simulink model "grzej_ret"  (R2019a)
settings: Solver=VariableStepAuto  StartTime=0.0  StopTime=TS  RelTol=1e-3
values from neighbouring files (symbols this model uses):
  cpw = 4175    [LAB1.m]    (also in LAB2.m; LAB3.m)
  Cvg1 = cpw * row * Vg    (= 60120)    [LAB3.m]
  Cvk = Cvg    (= 40080000)    [LAB2.m]    (also in LAB3.m = 4175000; bezp.m = 4163040.816; budynek_z_hydraulika_symulacja.m = 249782.44896; kociol_pokoj_skrypt.m = 4163040.816)
  Cvw1 = cpp * rop * Vp1    (= 108000)    [LAB3.m]
  Cvw2 = cpp * rop * Vp2    (= 129600)    [LAB3.m]
  delta_t = 25000    [LAB3.m]
  df1 = 0    [LAB3.m]
  df2 = 0    [LAB3.m]
  dfmk = 0    [LAB2.m]    (also in LAB3.m)
  dqk = 0    [LAB2.m]    (also in LAB3.m = 2200)
  dT = 0    [LAB3.m]
  f10 = fmg1    (= 0.059880239521)    [LAB3.m]
  f20 = fmg2    (= 0.0718562874251)    [LAB3.m]
  fmk0 = fmkN    (= 1000)    [LAB2.m]    (also in LAB3.m = 0.131736526946)
  Kcg1 = (cpw*fmg1*(TkzN-Tgp1N))/(Tgp1N-Twew1N)    (= 100)    [LAB3.m]
  Kcg2 = (cpw*fmg2*(TkzN-Tgp2N))/(Tgp2N-Twew2N)    (= 120)    [LAB3.m]
  Kcp = (3*4)/0.20    (= 60)    [LAB3.m]
  Kcw1 = (Kcg1*(Tgp1N-Twew1N)-Kcp*(Twew1N-Twew2N))/(Twew1N-TzewN)    (= 125)    [LAB3.m]
  Kcw2 = (Kcg2*(Tgp2N-Twew2N)-Kcp*(Twew1N-Twew2N))/(Twew2N-TzewN)    (= 150)    [LAB3.m]
  qk0 = qgN    (= 20000)    [LAB2.m]    (also in LAB3.m = 11000)
  t0 = 0.1*TS    (= 100000)    [LAB3.m]
  Tgp10 = x(3)    [LAB3.m]
  Tgp20 = x(4)    [LAB3.m]
  Tkp0 = (fmg1*Tgp10+fmg2*Tgp20)/(fmg1+fmg2)    [LAB3.m]    (also in bezp.m = 72.5; kociol_pokoj_skrypt.m = 70; pogoda.m = 72.5; pogodowa.m = 70)
  Tkz0 = TgzN    (= 90)    [LAB2.m]    (also in LAB3.m = x(5); bezp.m = 91.5; kociol_pokoj_skrypt.m = 92; pogoda.m = 91.5)
  Twew10 = x(1)    [LAB3.m]
  Twew20 = x(2)    [LAB3.m]
  Tzew0 = TzewN    (= -20)    [LAB1.m]    (also in LAB2.m; LAB3.m; bezp.m = -13; grzejnik_pi_skrypt.m)
settings Model: Creator=ASUS  LastModifiedBy=ASUS
settings SolverCC: MaxConsecutiveMinStep=10  ShapePreserveControl=EnableAll

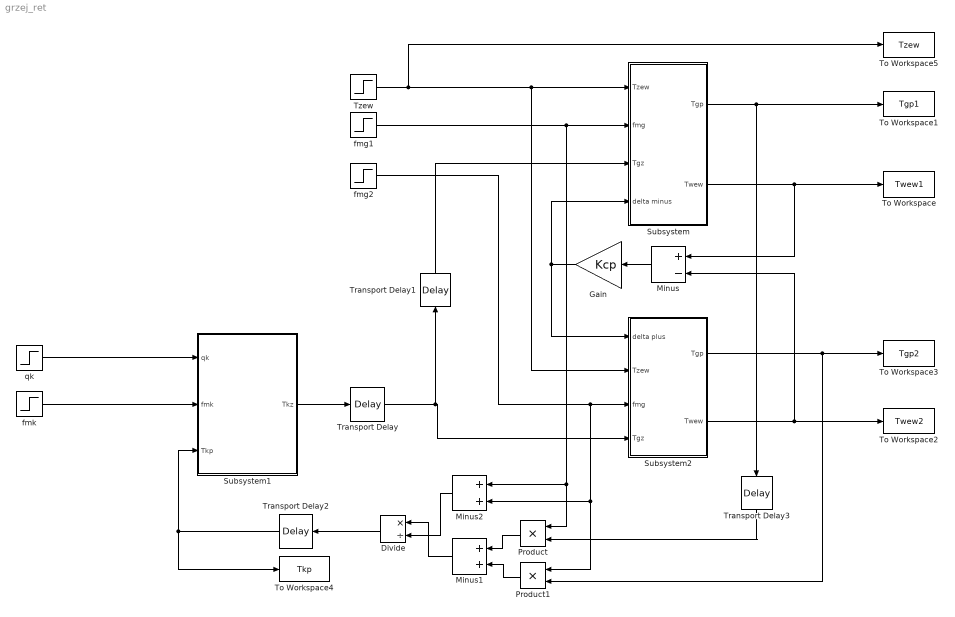
== system grzej_ret ==
  Divide : Product  Inputs=*/
  Gain : Gain  Gain=Kcp
  Minus : Sum  Inputs=+-
  Minus1 : Sum
  Minus2 : Sum
  Product : Product
  Product1 : Product
  Subsystem : Subsystem  mask{Kcg=Kcg1, Cvg=Cvg1, cpw=cpw, Kcw=Kcw1, Cvw=Cvw1, Tgp0=Tgp10, Twew0=Twew10}
  Subsystem1 : Subsystem  mask{Cvk=Cvk, cpw=cpw, Tkz0=Tkz0}
  Subsystem2 : Subsystem  mask{Kcg=Kcg2, Cvg=Cvg1, cpw=cpw, Kcw=Kcw2, Cvw=Cvw2, Tgp0=Tgp20, Twew0=Twew20}
  To Workspace : ToWorkspace  VariableName=Twew1  SampleTime=-1
  To Workspace1 : ToWorkspace  VariableName=Tgp1  SampleTime=-1
  To Workspace2 : ToWorkspace  VariableName=Twew2  SampleTime=-1
  To Workspace3 : ToWorkspace  VariableName=Tgp2  SampleTime=-1
  To Workspace4 : ToWorkspace  VariableName=Tkp  SampleTime=-1
  To Workspace5 : ToWorkspace  VariableName=Tzew  SampleTime=-1
  Transport Delay : TransportDelay  DelayTime=delta_t  InitialOutput=Tkz0
  Transport Delay1 : TransportDelay  DelayTime=delta_t  InitialOutput=Tkz0
  Transport Delay2 : TransportDelay  DelayTime=delta_t  InitialOutput=Tkp0
  Transport Delay3 : TransportDelay  DelayTime=delta_t  InitialOutput=Tgp10
  Tzew : Step  Time=t0  Before=Tzew0  After=Tzew0 + dT  SampleTime=0
  fmg1 : Step  Time=t0  Before=f10  After=f10+df1  SampleTime=0
  fmg2 : Step  Time=t0  Before=f20  After=f20+df2  SampleTime=0
  fmk : Step  Time=t0  Before=fmk0  After=fmk0 + dfmk  SampleTime=0
  qk : Step  Time=t0  Before=qk0  After=qk0+ dqk  SampleTime=0
  wires:
  Subsystem/1(Tgp) -> To Workspace1/1, Transport Delay3/1
  Subsystem/2(Twew) -> To Workspace/1, Minus/1
  Subsystem1/1(Tkz) -> Transport Delay/1
  Tzew/1 -> To Workspace5/1, Subsystem2/2(Tzew), Subsystem/1(Tzew)
  qk/1 -> Subsystem1/1(qk)
  fmk/1 -> Subsystem1/2(fmk)
  Subsystem2/2(Twew) -> Minus/2, To Workspace2/1
  Subsystem2/1(Tgp) -> Product1/2, To Workspace3/1
  Minus/1 -> Gain/1
  Gain/1 -> Subsystem/4("delta minus "), Subsystem2/1(delta plus)
  fmg1/1 -> Minus2/1, Product/1, Subsystem/2(fmg)
  fmg2/1 -> Minus2/2, Product1/1, Subsystem2/3(fmg)
  Product/1 -> Minus1/1
  Product1/1 -> Minus1/2
  Minus1/1 -> Divide/1
  Minus2/1 -> Divide/2
  Divide/1 -> Transport Delay2/1
  Transport Delay/1 -> Subsystem2/4(Tgz), Transport Delay1/1
  Transport Delay1/1 -> Subsystem/3(Tgz)
  Transport Delay3/1 -> Product/2
  Transport Delay2/1 -> Subsystem1/3(Tkp), To Workspace4/1

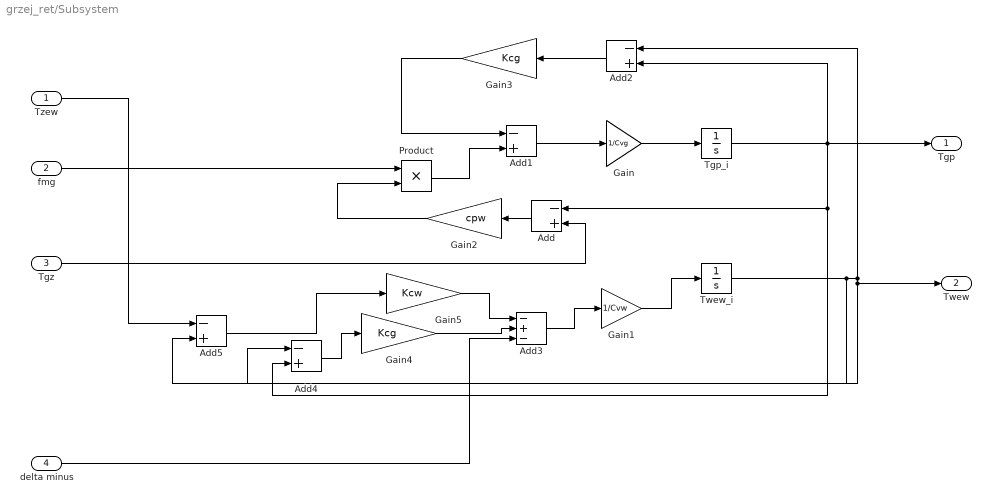
== system grzej_ret/Subsystem ==
  Tzew : Inport
  fmg : Inport  Port=2
  Tgz : Inport  Port=3
  "delta minus " : Inport  Port=4
  Add{,1..2,4..5} (5 alike) : Sum  Inputs=-+
  Add3 : Sum  Inputs=-+-
  Gain : Gain  Gain=1/Cvg
  Gain1 : Gain  Gain=1/Cvw
  Gain2 : Gain  Gain=cpw
  Gain3 : Gain  Gain=Kcg
  Gain4 : Gain  Gain=Kcg
  Gain5 : Gain  Gain=Kcw
  Product : Product
  Tgp_i : Integrator  InitialCondition=Tgp0
  Twew_i : Integrator  InitialCondition=Twew0
  Tgp : Outport
  Twew : Outport  Port=2
  wires:
  Add1/1 -> Gain/1
  Gain1/1 -> Twew_i/1
  Tgp_i/1 -> Tgp/1, Add2/2, Add4/2, Add/1
  Gain4/1 -> Add3/2
  Add2/1 -> Gain3/1
  Product/1 -> Add1/2
  Gain5/1 -> Add3/1
  Add4/1 -> Gain4/1
  Gain/1 -> Tgp_i/1
  Add5/1 -> Gain5/1
  Gain2/1 -> Product/2
  Tgz/1 -> Add/2
  Gain3/1 -> Add1/1
  Add3/1 -> Gain1/1
  Add/1 -> Gain2/1
  Twew_i/1 -> Add5/2, Twew/1, Add4/1, Add2/1
  fmg/1 -> Product/1
  Tzew/1 -> Add5/1
  "delta minus "/1 -> Add3/3

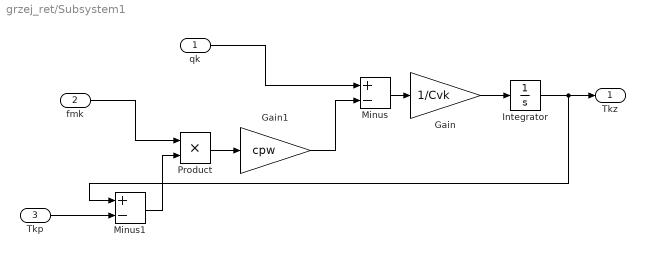
== system grzej_ret/Subsystem1 ==
  qk : Inport
  fmk : Inport  Port=2
  Tkp : Inport  Port=3
  Gain : Gain  Gain=1/Cvk
  Gain1 : Gain  Gain=cpw
  Integrator : Integrator  InitialCondition=Tkz0
  Minus : Sum  Inputs=+-
  Minus1 : Sum  Inputs=+-
  Product : Product
  Tkz : Outport
  wires:
  Integrator/1 -> Minus1/1, Tkz/1
  Gain/1 -> Integrator/1
  Minus/1 -> Gain/1
  qk/1 -> Minus/1
  Gain1/1 -> Minus/2
  Product/1 -> Gain1/1
  fmk/1 -> Product/1
  Tkp/1 -> Minus1/2
  Minus1/1 -> Product/2

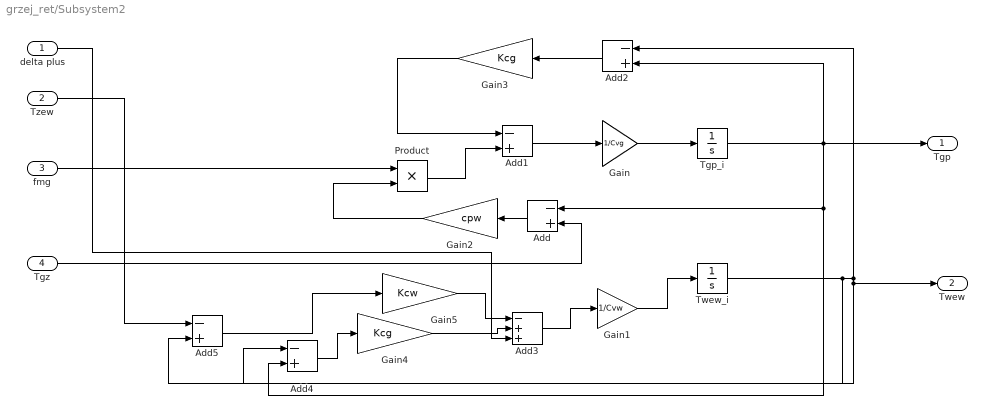
== system grzej_ret/Subsystem2 ==
  delta plus : Inport
  Tzew : Inport  Port=2
  fmg : Inport  Port=3
  Tgz : Inport  Port=4
  Add{,1..2,4..5} (5 alike) : Sum  Inputs=-+
  Add3 : Sum  Inputs=-++
  Gain : Gain  Gain=1/Cvg
  Gain1 : Gain  Gain=1/Cvw
  Gain2 : Gain  Gain=cpw
  Gain3 : Gain  Gain=Kcg
  Gain4 : Gain  Gain=Kcg
  Gain5 : Gain  Gain=Kcw
  Product : Product
  Tgp_i : Integrator  InitialCondition=Tgp0
  Twew_i : Integrator  InitialCondition=Twew0
  Tgp : Outport
  Twew : Outport  Port=2
  wires:
  Add1/1 -> Gain/1
  Gain1/1 -> Twew_i/1
  Tgp_i/1 -> Tgp/1, Add2/2, Add4/2, Add/1
  Gain4/1 -> Add3/2
  Add2/1 -> Gain3/1
  Product/1 -> Add1/2
  Gain5/1 -> Add3/1
  Add4/1 -> Gain4/1
  Gain/1 -> Tgp_i/1
  Add5/1 -> Gain5/1
  Gain2/1 -> Product/2
  Tgz/1 -> Add/2
  Gain3/1 -> Add1/1
  Add3/1 -> Gain1/1
  Add/1 -> Gain2/1
  Twew_i/1 -> Add5/2, Twew/1, Add4/1, Add2/1
  fmg/1 -> Product/1
  Tzew/1 -> Add5/1
  delta plus/1 -> Add3/3
